simulink model "Mod5counter"  (R2020b)
settings: Solver=VariableStepAuto  StartTime=0.0  StopTime=10.0  RelTol=1e-3
settings Model: Creator=Shivashis  LastModifiedBy=Shivashis

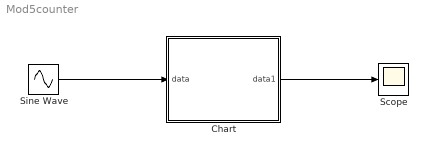
== system Mod5counter ==
  Chart : Stateflow chart  TreatAsAtomicUnit=on
  Scope : Scope
  Sine Wave : Sin  SampleTime=0
  wires:
  Sine Wave/1 -> Chart/1(data)
  Chart/1(data1) -> Scope/1

== stateflow chart Mod5counter/Chart ==
  state ?
  (default) -> ?
  data: data input; data1 output
